simulink model "Heli_Simulation"  (R2024a)
settings: Solver=ode1  StartTime=0.0  StopTime=30  FixedStep=.01  RelTol=1e-3  EnableMultiTasking=on
values from neighbouring files (symbols this model uses):
  D2R = pi/180.0    (= 0.0174532925199)    [Heli_Setup.m]
  ELEV_SLF = 24.25    [Heli_Setup.m]
  Kd = 0    [Heli_Setup.m]
  Kdt = 0    [Heli_Setup.m]
  Ki = 0    [Heli_Setup.m]
  Kit = 0    [Heli_Setup.m]
  Kp = 0    [Heli_Setup.m]
  Kpt = 0    [Heli_Setup.m]
  R2D = 180/pi    (= 57.2957795131)    [Heli_Setup.m]
  TRAV_SS = 90    [Heli_Setup.m]
libraries: cstblocks x2
Description:
  | Simulink(R) 3D Animation(TM) - Tutorial #3
  | 
  | Tutorial model to be used for 3D World Editor authoring example in the documentation.
  | After creating the virtual world according to the instructions in the documentation, include the VR block
  | in the model and connect B1, B2 coordinates and S scaling to corresponding nodes in
  | the virtual world.
settings Model: Creator=Danek  LastModifiedBy=danielmielnik
settings SolverCC: AlgebraicLoopSolver=TrustRegion
settings DataIOCC: LimitDataPoints=on  SaveFormat=Array  SignalLoggingSaveFormat=ModelDataLogs  SaveOutput=off  SaveTime=off  ReturnWorkspaceOutputs=off  SignalLoggingName=logsOut
settings OptimizationCC: BooleanDataType=off  ExpressionDepthLimit=2147483647  InitFltsAndDblsToZero=on  LifeSpan=inf
settings DebuggingCC: UnderspecifiedInitializationDetection=Classic  MergeDetectMultiDrivingBlocksExec=none  CheckExecutionContextPreStartOutputMsg=on  SignalResolutionControl=TryResolveAllWithWarning  MultiTaskDSMMsg=warning  MultiTaskCondExecSysMsg=none  FcnCallInpInsideContextMsg=warning  UnconnectedInputMsg=warning  UnconnectedOutputMsg=warning  UnconnectedLineMsg=warning  AllowSymbolicDim=off  StateNameClashWarn=warning  SFUnexpectedBacktrackingDiag=warning  SFNoUnconditionalDefaultTransitionDiag=warning  SFExecutionAtInitializationDiag=none  ArithmeticOperatorsInVariantConditions=warning
settings HardwareCC: ProdBitPerPointer=32  ProdBitPerSizeT=32  ProdBitPerPtrDiffT=32  ProdLargestAtomicFloat=None  ProdIntDivRoundTo=Undefined  ProdEndianess=Unspecified  ProdWordSize=32  ProdHWDeviceType=32-bit Generic  TargetBitPerLong=64  TargetBitPerPointer=64  TargetBitPerSizeT=64  TargetBitPerPtrDiffT=64  TargetLongLongMode=on  TargetIntDivRoundTo=Zero  TargetEndianess=LittleEndian  TargetWordSize=64  TargetHWDeviceType=MATLAB Host  ProdEqTarget=off
settings ModelReferenceCC: UpdateModelReferenceTargets=IfOutOfDate  EnableRefExpFcnMdlSchedulingChecks=on  PropagateSignalLabelsOutOfModel=off
settings SFSimCC: SimUseLocalCustomCode=off  CustomCodeUndefinedFunction=UseInterfaceOnly
settings RTWCC: RTWUseLocalCustomCode=off  GPUComputeCapability=3.5
settings CodeAppCC: StateflowObjectComments=on
settings GRTTargetCC: TargetFcnLib=ansi_tfl_tmw.mat  TargetLangStandard=C89/C90 (ANSI)  CombineOutputUpdateFcns=off  GRTInterface=on
settings ConfigComp: CovMetricSettings=d  CovSaveCumulativeToWorkspaceVar=on  CovSaveSingleToWorkspaceVar=on  CovExternalEMLEnable=off

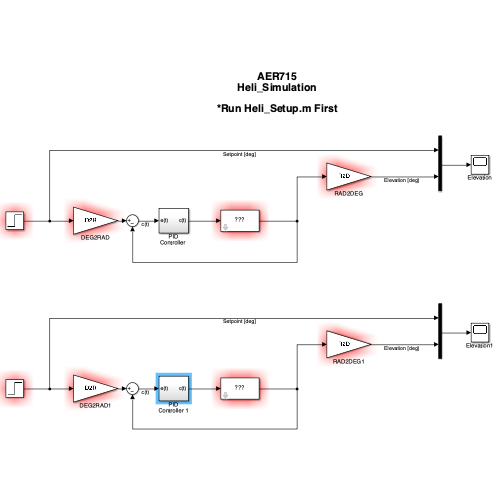
[thumbnail: Simulink's stored preview of the top-level diagram]
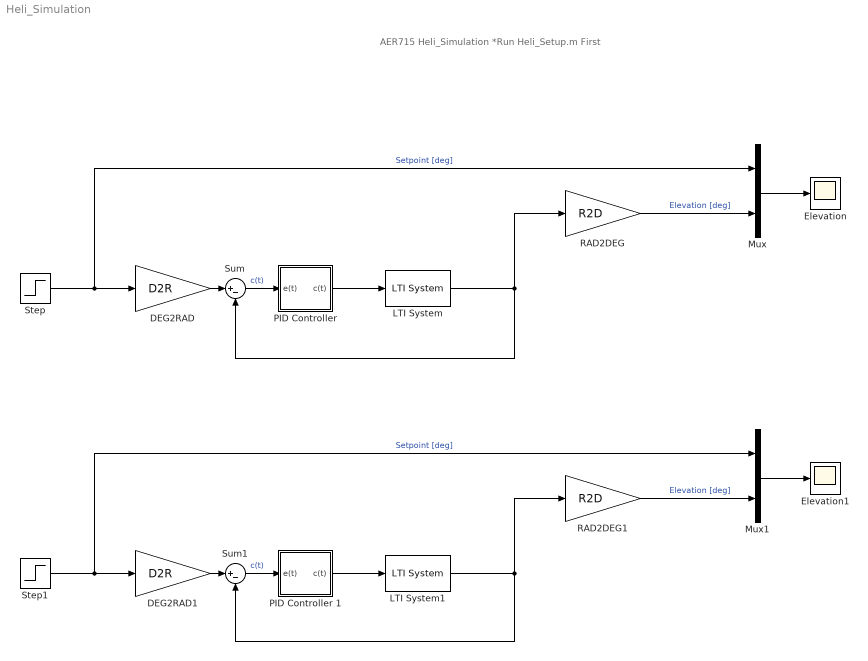
== system Heli_Simulation ==
  note: AER715
      | Heli_Simulation
      |
      | *Run Heli_Setup.m First
  " PID Controller " : Subsystem
  " PID Controller 1" : Subsystem
  DEG2RAD : Gain  Gain=D2R
  DEG2RAD1 : Gain  Gain=D2R
  Elevation : Scope
  Elevation1 : Scope
  LTI System : cstblocks/LTI System  sys=G1_elev1  IC=[]  PadeOrder=0
  LTI System1 : cstblocks/LTI System  sys=G1_elev1  IC=[]  PadeOrder=0
  Mux : Mux  Inputs=2
  Mux1 : Mux  Inputs=2
  RAD2DEG : Gain  Gain=R2D
  RAD2DEG1 : Gain  Gain=R2D
  Step : Step  After=ELEV_SLF  SampleTime=.01
  Step1 : Step  Time=25  After=TRAV_SS  SampleTime=.01
  Sum : Sum  Inputs=|+-
  Sum1 : Sum  Inputs=|+-
  wires:
  LTI System/1 -> Sum/2, RAD2DEG/1
  DEG2RAD/1 -> Sum/1
  Sum/1 -> " PID Controller "/1(e(t))  "c(t)"
  " PID Controller "/1(c(t)) -> LTI System/1
  RAD2DEG/1 -> Mux/2  "Elevation [deg]"
  Mux/1 -> Elevation/1
  Step/1 -> DEG2RAD/1, Mux/1  "Setpoint [deg]"
  DEG2RAD1/1 -> Sum1/1
  " PID Controller 1"/1(c(t)) -> LTI System1/1
  LTI System1/1 -> Sum1/2, RAD2DEG1/1
  RAD2DEG1/1 -> Mux1/2  "Elevation [deg]"
  Mux1/1 -> Elevation1/1
  Sum1/1 -> " PID Controller 1"/1(e(t))  "c(t)"
  Step1/1 -> DEG2RAD1/1, Mux1/1  "Setpoint [deg]"

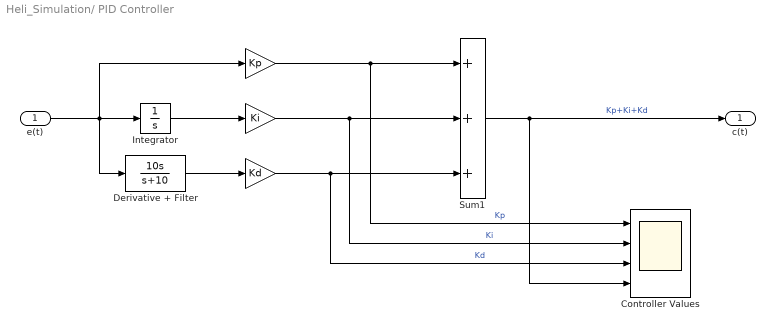
== system Heli_Simulation/ PID Controller  ==
  e(t) : Inport
  " " : Gain  Gain=Kp
  "  " : Gain  Gain=Ki
  "   " : Gain  Gain=Kd
  Controller Values : Scope  NumInputPorts=4
  Derivative + Filter : TransferFcn  Numerator=[10 0]  Denominator=[1 10]
  Integrator : Integrator  UpperSaturationLimit=30  LowerSaturationLimit=-30
  Sum1 : Sum  Inputs=+++
  c(t) : Outport
  wires:
  " "/1 -> Sum1/1, Controller Values/1  "Kp"
  Sum1/1 -> c(t)/1, Controller Values/4  "Kp+Ki+Kd"
  "  "/1 -> Sum1/2, Controller Values/2  "Ki"
  "   "/1 -> Sum1/3, Controller Values/3  "Kd"
  Derivative + Filter/1 -> "   "/1
  Integrator/1 -> "  "/1
  e(t)/1 -> Integrator/1, Derivative + Filter/1, " "/1

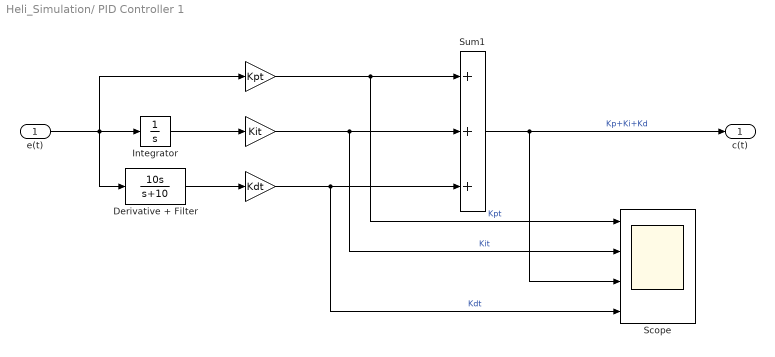
== system Heli_Simulation/ PID Controller 1 ==
  e(t) : Inport
  " " : Gain  Gain=Kpt
  "  " : Gain  Gain=Kit
  "   " : Gain  Gain=Kdt
  Derivative + Filter : TransferFcn  Numerator=[10 0]  Denominator=[1 10]
  Integrator : Integrator  UpperSaturationLimit=30  LowerSaturationLimit=-30
  Scope : Scope  NumInputPorts=4
  Sum1 : Sum  Inputs=+++
  c(t) : Outport
  wires:
  " "/1 -> Scope/1, Sum1/1  "Kpt"
  Sum1/1 -> Scope/3, c(t)/1  "Kp+Ki+Kd"
  "  "/1 -> Scope/2, Sum1/2  "Kit"
  "   "/1 -> Scope/4, Sum1/3  "Kdt"
  Derivative + Filter/1 -> "   "/1
  Integrator/1 -> "  "/1
  e(t)/1 -> Integrator/1, Derivative + Filter/1, " "/1
